simulink model "Model_3"  (R2019b)
settings: Solver=ode15s  StartTime=0.0  StopTime=35  MaxStep=0.005  RelTol=1e-3
model workspace (MATLAB code in the model file):
  | ms = 135;
  | mf = 5;
  | mr = 10;
  | m = ms + (mf + mr);
  | a = 0.7;
  | b = 0.7;
  | Cd = 0.8;
  | Af = 1;
  | h_cg = 0.5;
  | kf = 10000;
  | kr = 15000;
  | cf = 5000;
  | cr = 5000;
  | I = 500;
  | kt = 175000;
values from neighbouring files (symbols this model uses):
  GR = 6.5    [Model_1_timeto40.m]    (also in Model_1_timeto60.m; Model_3_topspeed.m)
  Pmax = P(i,j)    [Model_1_timeto40.m]    (also in Model_1_timeto60.m; Model_3_topspeed.m = P(i))
libraries: autolibshared x2
(part 1 of 3)
settings Model: Creator=Barath Krishna S  LastModifiedBy=Barath Krishna S
settings DataIOCC: SaveFormat=Array  SaveOutput=off  SaveState=on  SignalLogging=off  DSMLogging=off

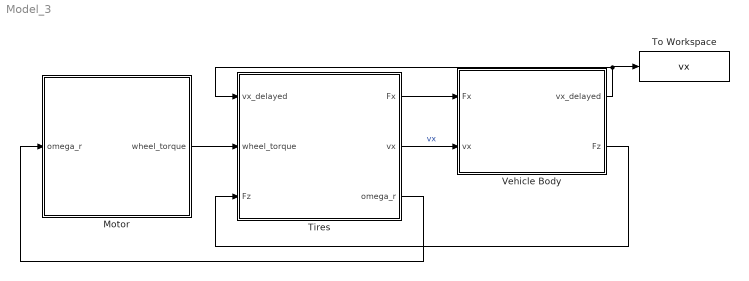
== system Model_3 ==
  Motor : Subsystem
  Tires : Subsystem
  To Workspace : ToWorkspace  VariableName=vx  SampleTime=-1
      settings: MaxDataPoints=1
  Vehicle Body : Subsystem
  wires:
  Tires/2(vx) -> Vehicle Body/2(vx)  "vx"
  Tires/3(omega_r) -> Motor/1(omega_r)
  Tires/1(Fx) -> Vehicle Body/1(Fx)
  Vehicle Body/1(vx_delayed) -> To Workspace/1, Tires/1(vx_delayed)
  Vehicle Body/2(Fz) -> Tires/3(Fz)
  Motor/1(wheel_torque) -> Tires/2(wheel_torque)

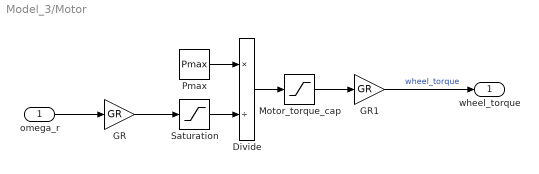
== system Model_3/Motor ==
  omega_r : Inport
  Divide : Product  Inputs=*/
  GR : Gain  Gain=GR
  GR1 : Gain  Gain=GR
  Motor_torque_cap : Saturate  UpperLimit=26  LowerLimit=0
  Pmax : Constant  Value=Pmax
  Saturation : Saturate  UpperLimit=inf  LowerLimit=0.001
  wheel_torque : Outport
  wires:
  Pmax/1 -> Divide/1
  Saturation/1 -> Divide/2
  Divide/1 -> Motor_torque_cap/1
  omega_r/1 -> GR/1
  GR/1 -> Saturation/1
  Motor_torque_cap/1 -> GR1/1
  GR1/1 -> wheel_torque/1  "wheel_torque"
